simulink model "eclipse_target_lqri"  (Simulink 7.6)
settings: Solver=FixedStepDiscrete  StartTime=0.0  StopTime=inf  FixedStep=Ts  RelTol=1e-3
PreLoadFcn:
  | load_waypoints
values from neighbouring files (symbols this model uses):
  g = 9.8065    [kostas_malakies.mat]    (also in kostas_malakies2.mat; load_PMModel.m = 9.81; main.m; main_last.m)
  mass = 0.66    [kostas_malakies.mat]    (also in kostas_malakies2.mat; load_PMModel.m = 0.687; main_last.m)
  Ts = 0.02    [kostas_malakies.mat]    (also in kostas_malakies2.mat; main.m; main_last.m; matlab.mat = 0.08)
undefined symbols (not defined in the file or in its folder): DiscIntNeverNeededParam
libraries: Hquad_control_LIB_LQRI x13, Hqaud_model_LIB_SI x1, idelinklib_tgtpref x1, simulink x1
settings Model: Creator=janosch  LastModifiedBy=burrimi  SimulationMode=external
settings DataIOCC: SaveOutput=off  SaveTime=off
settings OptimizationCC: OptimizeModelRefInitCode=on  LifeSpan=1
settings DebuggingCC: ParameterPrecisionLossMsg=none
settings HardwareCC: ProdIntDivRoundTo=Zero  ProdEndianess=LittleEndian  ProdHWDeviceType=Intel Pentium
settings RTWCC: SystemTargetFile=idelink_ert.tlc  GenerateMakefile=off  TemplateMakefile=idelink_ert.tmf  Description=Embedded IDE Link ERT  ProcessScript=idelink_ert_make_rtw_hook
settings CodeAppCC: IgnoreCustomStorageClasses=off
settings ERTFactory: TargetFcnLib=ansi_tfl_table_tmw.mat  TargetFunctionLibrary=ANSI_C  UtilityFuncGeneration=Auto  ERTMultiwordTypeDef=System defined  ERTCodeCoverageTool=None  ERTMultiwordLength=256  MultiwordLength=2048  GenerateFullHeader=on  GenerateSampleERTMain=off  GenerateTestInterfaces=off  IsPILTarget=off  ModelReferenceCompliant=on  ParMdlRefBuildCompliant=off  CompOptLevelCompliant=off  IncludeMdlTerminateFcn=on  GeneratePreprocessorConditionals=Disable all  CombineOutputUpdateFcns=on  CombineSignalStateStructs=off  SuppressErrorStatus=off  ERTFirstTimeCompliant=off  IncludeFileDelimiter=Auto  ERTCustomFileBanners=on  SupportAbsoluteTime=on  LogVarNameModifier=rt_  MatFileLogging=off  MultiInstanceERTCode=off  SupportNonFinite=on  SupportComplex=on  PurelyIntegerCode=off  SupportContinuousTime=off  SupportNonInlinedSFcns=on  SupportVariableSizeSignals=off  EnableShiftOperators=on  ParenthesesLevel=Nominal  PortableWordSizes=off  ModelStepFunctionPrototypeControlCompliant=on  CPPClassGenCompliant=off  AutosarCompliant=off  GenerateErtSFunction=off  CreateSILPILBlock=None  GenerateASAP2=off  ExtMode=on  ExtModeTransport=0  ExtModeStaticAlloc=off  ExtModeStaticAllocSize=1000000  ExtModeTesting=off  ExtModeMexFile=ext_comm  ExtModeIntrfLevel=Level1  InlinedParameterPlacement=Hierarchical  TargetOS=BareBoardExample  MultiInstanceErrorCode=Error  RateGroupingCode=on  RootIOFormat=Individual arguments  RTWCAPISignals=off  RTWCAPIParams=off  RTWCAPIStates=off  ERTSrcFileBannerTemplate=ert_code_template.cgt  ERTHdrFileBannerTemplate=ert_code_template.cgt  ERTDataSrcFileTemplate=ert_code_template.cgt  ERTDataHdrFileTemplate=ert_code_template.cgt  ERTCustomFileTemplate=example_file_process.tlc  CoverageDialogOpen=off  ModuleNamingRule=Unspecified  SignalDisplayLevel=10  ParamTuneLevel=10  GlobalDataDefinition=Auto  DataDefinitionFile=global.c  GlobalDataReference=Auto  ERTFilePackagingFormat=Modular  DataReferenceFile=global.h  GRTInterface=off  PreserveExpressionOrder=off  PreserveIfCondition=off  ConvertIfToSwitch=off  PreserveExternInFcnDecls=on  EnableUserReplacementTypes=off  MemSecPackage=--- None ---  MemSecDataConstants=Default  MemSecDataIO=Default  MemSecDataInternal=Default  MemSecDataParameters=Default  MemSecFuncInitTerm=Default  MemSecFuncExecute=Default  AdaptorName=Eclipse  exportIDEObj=on  ideObjName=IDE_Obj  oldideObjName=IDE_Obj  ideObjTimeout=50  oldideObjTimeout=50  ideObjBuildTimeout=1000  oldideObjBuildTimeout=1000  ProfileGenCode=off  profileBy=Tasks  ProfileNumSamples=100  InlineDSPBlks=off  projectOptions=Custom  debugCompilerOptions="-g -D\"_DEBUG\""  releaseCompilerOptions=-O2  getCompilerOptions=off  resetCompilerOptions=off  debugLinkerOptions=-lm  releaseLinkerOptions=-lm  customLinkerOptions=-lm  linkerOptionsStr=-lm  getLinkerOptions=off  resetLinkerOptions=off  systemStackSize=512  systemHeapSize=512  buildFormat=Project  buildAction=Build  overrunNotificationMethod=None  overrunNotificationFcn=myfunction  oldoverrunNotificationFcn=myfunction  configurePIL=off  configPILBlockAction=Create_PIL_block_build_and_download  DiagnosticActions=warning

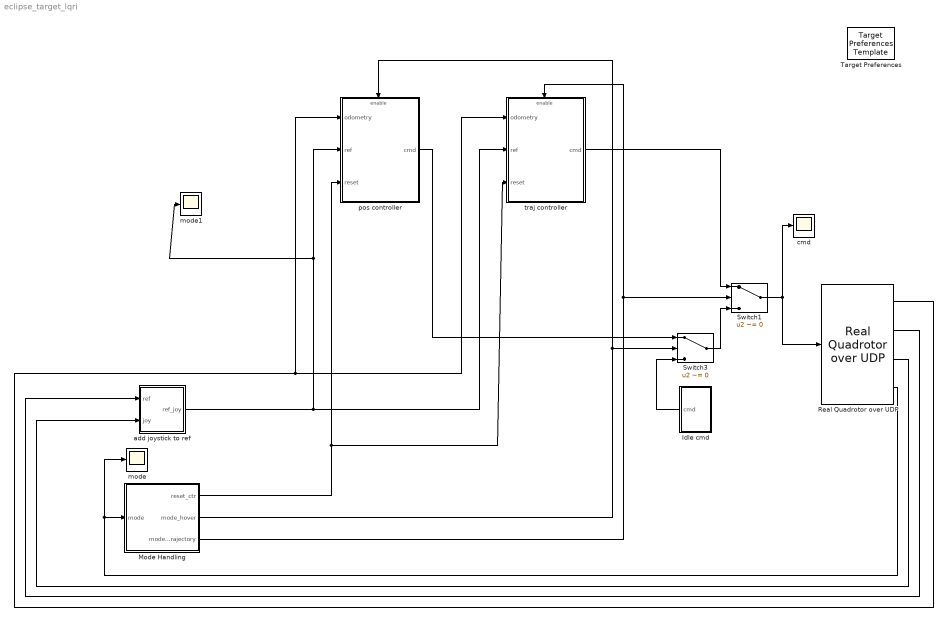
== system eclipse_target_lqri ==
  Idle cmd : Subsystem
  Mode Handling : Subsystem
  Real Quadrotor over UDP : Hqaud_model_LIB_SI/Real Quadrotor over UDP  SystemSampleTime=-1
  Switch1 : Switch  Criteria=u2 ~= 0
  Switch3 : Switch  Criteria=u2 ~= 0
  Target Preferences : idelinklib_tgtpref/Target Preferences Template  Tag=eclipseidetgtpref  SystemSampleTime=-1  library=off
  add joystick to ref : Subsystem
  cmd : Scope
      settings: YMin=-0.5  YMax=7  SaveName=ScopeData4
  mode : Scope
      settings: YMin=0  YMax=6  SaveName=ScopeData6
  mode1 : Scope
      settings: YMin=-2  YMax=2  SaveName=ScopeData7
  pos controller : Subsystem  AncestorBlock=Hquad_control_LIB_LQRI/pos controller
  traj controller : Subsystem  AncestorBlock=Hquad_control_LIB_LQRI/traj controller
  wires:
  Mode Handling/1(reset_ctr) -> pos controller/3(reset), traj controller/3(reset)
  Mode Handling/2(mode_hover) -> Switch3/2, pos controller/Enable
  Idle cmd/1(cmd) -> Switch3/3
  pos controller/1(cmd) -> Switch3/1
  Mode Handling/3(mode_trajectory) -> Switch1/2, traj controller/Enable
  Switch3/1 -> Switch1/3
  Switch1/1 -> cmd/1, Real Quadrotor over UDP/1
  traj controller/1(cmd) -> Switch1/1
  Real Quadrotor over UDP/3 -> add joystick to ref/2(joy)
  add joystick to ref/1(ref_joy) -> mode1/1, pos controller/2(ref), traj controller/2(ref)
  Real Quadrotor over UDP/2 -> add joystick to ref/1(ref)
  Real Quadrotor over UDP/1 -> pos controller/1(odometry), traj controller/1(odometry)
  Real Quadrotor over UDP/4 -> Mode Handling/1(mode), mode/1

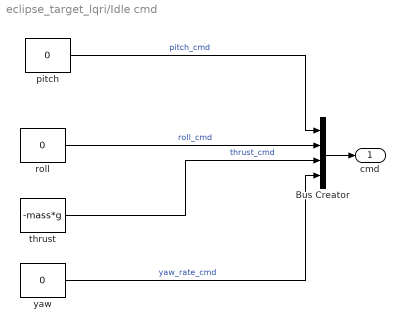
== system eclipse_target_lqri/Idle cmd ==
  Bus Creator : BusCreator
  pitch : Constant  Value=0
  roll : Constant  Value=0
  thrust : Constant  Value=-mass*g
  yaw : Constant  Value=0
  cmd : Outport
  wires:
  roll/1 -> Bus Creator/2  "roll_cmd"
  pitch/1 -> Bus Creator/1  "pitch_cmd"
  Bus Creator/1 -> cmd/1
  thrust/1 -> Bus Creator/3  "thrust_cmd"
  yaw/1 -> Bus Creator/4  "yaw_rate_cmd"

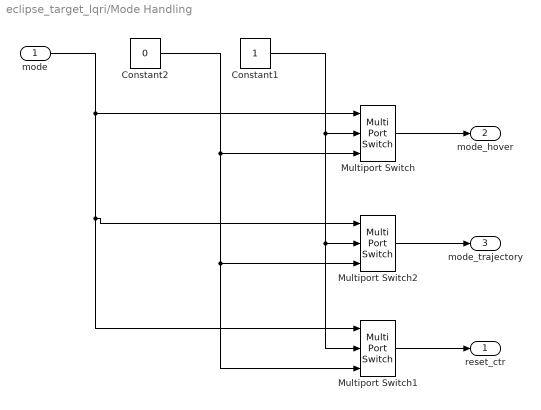
== system eclipse_target_lqri/Mode Handling ==
  mode : Inport
  Constant1 : Constant
  Constant2 : Constant  Value=0
  Multiport Switch : MultiPortSwitch  DataPortOrder=Specify indices  Inputs=2  DataPortIndices={[1,2,3],0}  zeroidx=off
  Multiport Switch1 : MultiPortSwitch  DataPortOrder=Specify indices  Inputs=2  DataPortIndices={[10],0}  zeroidx=off
  Multiport Switch2 : MultiPortSwitch  DataPortOrder=Specify indices  Inputs=2  DataPortIndices={[4],0}  zeroidx=off
  reset_ctr : Outport
  mode_hover : Outport  Port=2
  mode_trajectory : Outport  Port=3
  wires:
  Constant1/1 -> Multiport Switch/2, Multiport Switch1/2, Multiport Switch2/2
  Constant2/1 -> Multiport Switch/3, Multiport Switch1/3, Multiport Switch2/3
  Multiport Switch1/1 -> reset_ctr/1
  mode/1 -> Multiport Switch/1, Multiport Switch1/1, Multiport Switch2/1
  Multiport Switch/1 -> mode_hover/1
  Multiport Switch2/1 -> mode_trajectory/1

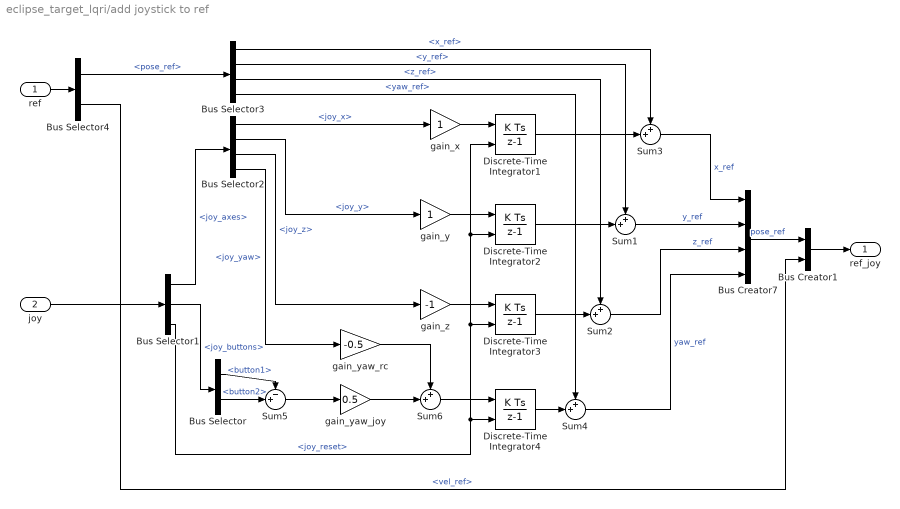
== system eclipse_target_lqri/add joystick to ref ==
  ref : Inport
  joy : Inport  Port=2
  Bus Creator1 : BusCreator  Inputs=2
  Bus Creator7 : BusCreator
  Bus Selector : BusSelector  OutputSignals=button1,button2
  Bus Selector1 : BusSelector  OutputSignals=joy_axes,joy_buttons,joy_reset
  Bus Selector2 : BusSelector  OutputSignals=joy_x,joy_y,joy_z,joy_yaw
  Bus Selector3 : BusSelector  OutputSignals=x_ref,y_ref,z_ref,yaw_ref
  Bus Selector4 : BusSelector  OutputSignals=pose_ref,vel_ref
  Discrete-Time Integrator{1..4} (4 alike) : DiscreteIntegrator  ExternalReset=rising  SampleTime=Ts  ICPrevOutput=DiscIntNeverNeededParam  ICPrevScaledInput=DiscIntNeverNeededParam
  Sum{1..4,6} (5 alike) : Sum  Inputs=++|
  Sum5 : Sum  Inputs=-+|
  gain_x : Gain
  gain_y : Gain
  gain_yaw_joy : Gain  Gain=0.5
  gain_yaw_rc : Gain  Gain=-0.5
  gain_z : Gain  Gain=-1
  ref_joy : Outport
  wires:
  Bus Selector2/1 -> gain_x/1  "<joy_x>"
  Bus Selector2/2 -> gain_y/1  "<joy_y>"
  Bus Selector2/3 -> gain_z/1  "<joy_z>"
  gain_x/1 -> Discrete-Time Integrator1/1
  gain_y/1 -> Discrete-Time Integrator2/1
  gain_z/1 -> Discrete-Time Integrator3/1
  Bus Selector3/1 -> Sum3/1  "<x_ref>"
  Bus Selector3/2 -> Sum1/1  "<y_ref>"
  Bus Selector3/3 -> Sum2/1  "<z_ref>"
  Discrete-Time Integrator1/1 -> Sum3/2
  Discrete-Time Integrator2/1 -> Sum1/2
  Discrete-Time Integrator3/1 -> Sum2/2
  Sum4/1 -> Bus Creator7/4  "yaw_ref"
  Sum2/1 -> Bus Creator7/3  "z_ref"
  Sum1/1 -> Bus Creator7/2  "y_ref"
  Sum3/1 -> Bus Creator7/1  "x_ref"
  Bus Selector1/2 -> Bus Selector/1  "<joy_buttons>"
  Bus Selector1/3 -> Discrete-Time Integrator3/2, Discrete-Time Integrator1/2, Discrete-Time Integrator2/2, Discrete-Time Integrator4/2  "<joy_reset>"
  Bus Selector/1 -> Sum5/1  "<button1>"
  Bus Selector/2 -> Sum5/2  "<button2>"
  Discrete-Time Integrator4/1 -> Sum4/2
  Bus Selector3/4 -> Sum4/1  "<yaw_ref>"
  joy/1 -> Bus Selector1/1
  Bus Selector1/1 -> Bus Selector2/1  "<joy_axes>"
  ref/1 -> Bus Selector4/1
  Bus Creator1/1 -> ref_joy/1
  Sum5/1 -> gain_yaw_joy/1
  Sum6/1 -> Discrete-Time Integrator4/1
  Bus Selector2/4 -> gain_yaw_rc/1  "<joy_yaw>"
  gain_yaw_rc/1 -> Sum6/1
  gain_yaw_joy/1 -> Sum6/2
  Bus Creator7/1 -> Bus Creator1/1  "pose_ref"
  Bus Selector4/1 -> Bus Selector3/1  "<pose_ref>"
  Bus Selector4/2 -> Bus Creator1/2  "<vel_ref>"

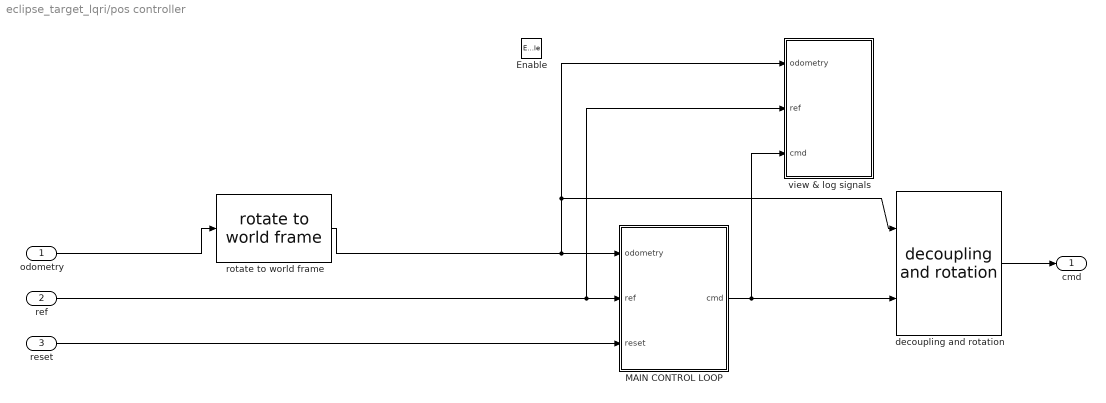
== system eclipse_target_lqri/pos controller ==
  odometry : Inport
  ref : Inport  Port=2
  reset : Inport  Port=3
  Enable : EnablePort  StatesWhenEnabling=reset
  MAIN CONTROL LOOP : Subsystem  AncestorBlock=Hquad_control_LIB_LQRI/MAIN CONTROL LOOP  TreatAsAtomicUnit=on
  decoupling and rotation : Hquad_control_LIB_LQRI/decoupling and rotation  Priority=3  SystemSampleTime=-1
  rotate to world frame : Hquad_control_LIB_LQRI/rotate to world frame  Priority=1  SystemSampleTime=-1
  view & log signals : Subsystem  AncestorBlock=Hquad_control_LIB_LQRI/view & log signals
  cmd : Outport
  wires:
  ref/1 -> MAIN CONTROL LOOP/2(ref), view & log signals/2(ref)
  reset/1 -> MAIN CONTROL LOOP/3(reset)
  odometry/1 -> rotate to world frame/1
  rotate to world frame/1 -> view & log signals/1(odometry), decoupling and rotation/1, MAIN CONTROL LOOP/1(odometry)
  MAIN CONTROL LOOP/1(cmd) -> view & log signals/3(cmd), decoupling and rotation/2
  decoupling and rotation/1 -> cmd/1

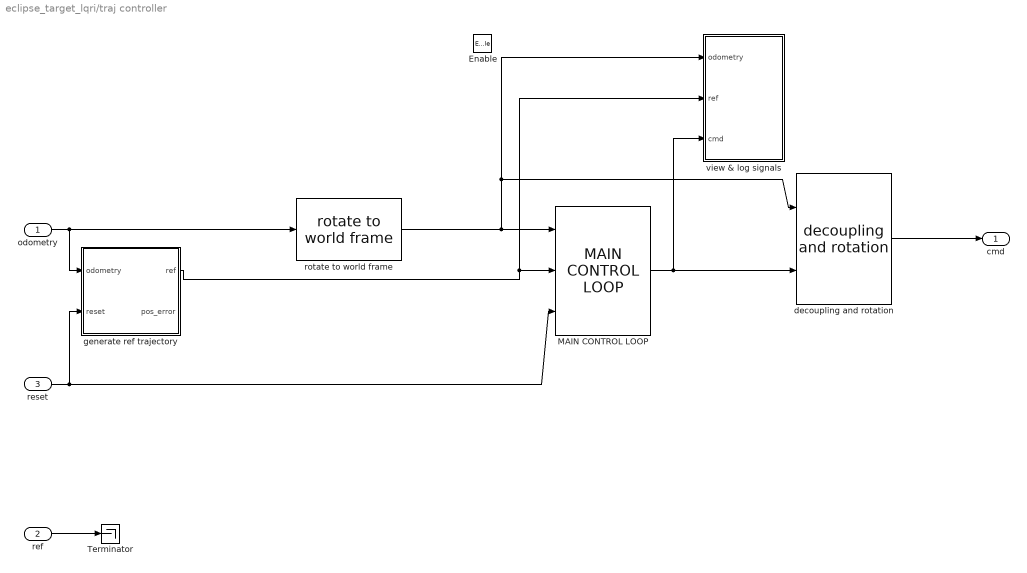
== system eclipse_target_lqri/traj controller ==
  odometry : Inport
  ref : Inport  Port=2
  reset : Inport  Port=3
  Enable : EnablePort  StatesWhenEnabling=reset
  MAIN CONTROL LOOP : Hquad_control_LIB_LQRI/MAIN CONTROL LOOP  SystemSampleTime=-1
  Terminator : Terminator
  decoupling and rotation : Hquad_control_LIB_LQRI/decoupling and rotation  Priority=3  SystemSampleTime=-1
  generate ref trajectory : Subsystem  AncestorBlock=Hquad_control_LIB_LQRI/generate ref trajectory
  rotate to world frame : Hquad_control_LIB_LQRI/rotate to world frame  Priority=1  SystemSampleTime=-1
  view & log signals : Subsystem  AncestorBlock=Hquad_control_LIB_LQRI/view & log signals
  cmd : Outport
  wires:
  generate ref trajectory/1(ref) -> MAIN CONTROL LOOP/2, view & log signals/2(ref)
  reset/1 -> MAIN CONTROL LOOP/3, generate ref trajectory/2(reset)
  ref/1 -> Terminator/1
  odometry/1 -> rotate to world frame/1, generate ref trajectory/1(odometry)
  rotate to world frame/1 -> view & log signals/1(odometry), decoupling and rotation/1, MAIN CONTROL LOOP/1
  MAIN CONTROL LOOP/1 -> view & log signals/3(cmd), decoupling and rotation/2
  decoupling and rotation/1 -> cmd/1

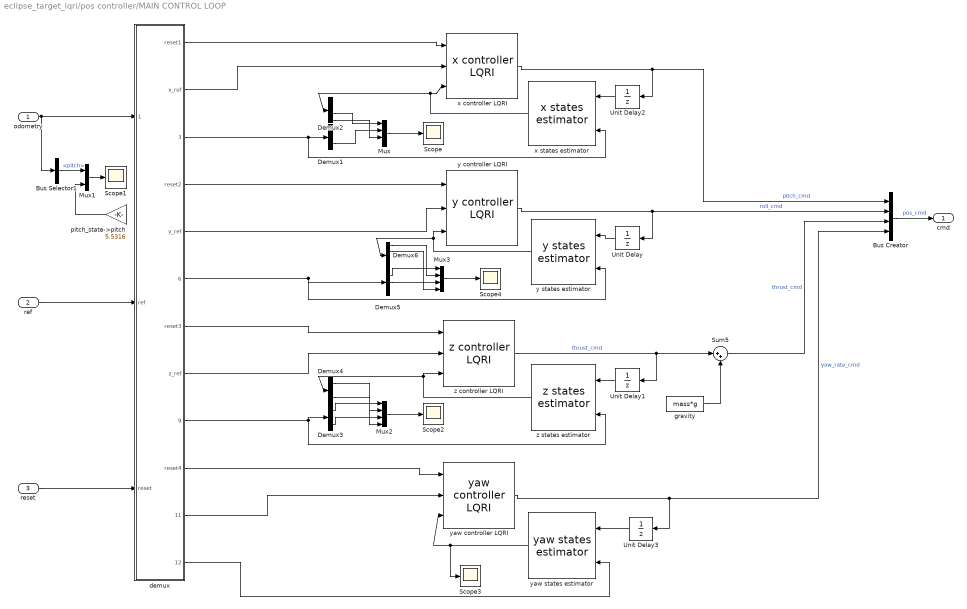
== system eclipse_target_lqri/pos controller/MAIN CONTROL LOOP ==
  odometry : Inport
  ref : Inport  Port=2
  reset : Inport  Port=3
  Bus Creator : BusCreator
  Bus Selector1 : BusSelector  OutputSignals=rpy.pitch
  Demux1 : Demux  Outputs=3
  Demux2 : Demux
  Demux3 : Demux  Outputs=2
  Demux4 : Demux  Outputs=2
  Demux5 : Demux  Outputs=3
  Demux6 : Demux
  Mux : Mux
  Mux1 : Mux  Inputs=2
  Mux2 : Mux
  Mux3 : Mux
  Scope{,1..4} (5 alike) : Scope
      Scope settings: TimeRange=8.564360869565219  YMin=-50  YMax=2.5  SaveName=ScopeData13
      Scope1 settings: YMin=-0.4  YMax=1.4  SaveName=ScopeData14
      Scope2 settings: YMin=-1.5  YMax=0.4  SaveName=ScopeData15
      Scope3 settings: YMin=-0.03  YMax=0.09  SaveName=ScopeData16
      Scope4 settings: TimeRange=8.564360869565219  YMin=-0.2  YMax=2  SaveName=ScopeData4
  Sum5 : Sum  Inputs=|++
  Unit Delay{,1..3} (4 alike) : UnitDelay  SampleTime=Ts
  demux : Subsystem
  gravity : Constant  Value=mass*g
  pitch_state->pitch : Gain  Gain=5.5316
  "x controller LQRI  " : Hquad_control_LIB_LQRI/x controller LQRI    SystemSampleTime=-1
  x states estimator : Hquad_control_LIB_LQRI/x states estimator  SystemSampleTime=-1
  y controller LQRI : Hquad_control_LIB_LQRI/y controller LQRI  SystemSampleTime=-1
  y states estimator : Hquad_control_LIB_LQRI/y states estimator  SystemSampleTime=-1
  yaw controller LQRI : Hquad_control_LIB_LQRI/yaw controller LQRI  SystemSampleTime=-1
  yaw states estimator : Hquad_control_LIB_LQRI/yaw states estimator  SystemSampleTime=-1
  z controller LQRI : Hquad_control_LIB_LQRI/z controller LQRI  SystemSampleTime=-1
  z states estimator : Hquad_control_LIB_LQRI/z states estimator  SystemSampleTime=-1
  cmd : Outport
  wires:
  Unit Delay3/1 -> yaw states estimator/1
  Sum5/1 -> Bus Creator/3  "thrust_cmd"
  demux/11(yaw_ref) -> yaw controller LQRI/2
  demux/9(z_states_meas) -> z states estimator/2, Demux3/1
  demux/6(y_states_meas) -> y states estimator/2, Demux5/1
  demux/3(x_states_meas) -> x states estimator/2, Demux1/1
  Bus Creator/1 -> cmd/1  "pos_cmd"
  demux/10(reset4) -> yaw controller LQRI/1
  demux/1(reset1) -> "x controller LQRI  "/1
  reset/1 -> demux/3(reset)
  ref/1 -> demux/2(ref)
  odometry/1 -> demux/1(odometry), Bus Selector1/1
  yaw controller LQRI/1 -> Unit Delay3/1, Bus Creator/4  "yaw_rate_cmd"
  demux/12(yaw_states_meas) -> yaw states estimator/2
  Unit Delay2/1 -> x states estimator/1
  Unit Delay1/1 -> z states estimator/1
  Unit Delay/1 -> y states estimator/1
  demux/2(x_ref) -> "x controller LQRI  "/2
  x states estimator/1 -> "x controller LQRI  "/3, Demux2/1
  y states estimator/1 -> y controller LQRI/3, Demux6/1
  "x controller LQRI  "/1 -> Unit Delay2/1, Bus Creator/1  "pitch_cmd"
  y controller LQRI/1 -> Unit Delay/1, Bus Creator/2  "roll_cmd"
  z states estimator/1 -> z controller LQRI/3, Demux4/1
  Mux/1 -> Scope/1
  Mux1/1 -> Scope1/1
  Bus Selector1/1 -> Mux1/1  "<pitch>"
  pitch_state->pitch/1 -> Mux1/2
  Mux2/1 -> Scope2/1
  Demux3/1 -> Mux2/1
  Demux4/1 -> Mux2/2
  Demux3/2 -> Mux2/3
  z controller LQRI/1 -> Unit Delay1/1, Sum5/1  "thrust_cmd"
  yaw states estimator/1 -> yaw controller LQRI/3, Scope3/1
  gravity/1 -> Sum5/2
  demux/5(y_ref) -> y controller LQRI/2
  demux/4(reset2) -> y controller LQRI/1
  Mux3/1 -> Scope4/1
  Demux5/1 -> Mux3/1
  Demux6/1 -> Mux3/2
  Demux5/2 -> Mux3/3
  Demux6/2 -> Mux3/4
  Demux4/2 -> Mux2/4
  demux/8(z_ref) -> z controller LQRI/2
  demux/7(reset3) -> z controller LQRI/1
  Demux2/3 -> Mux/1
  Demux1/3 -> Mux/2
  Demux2/4 -> Mux/3

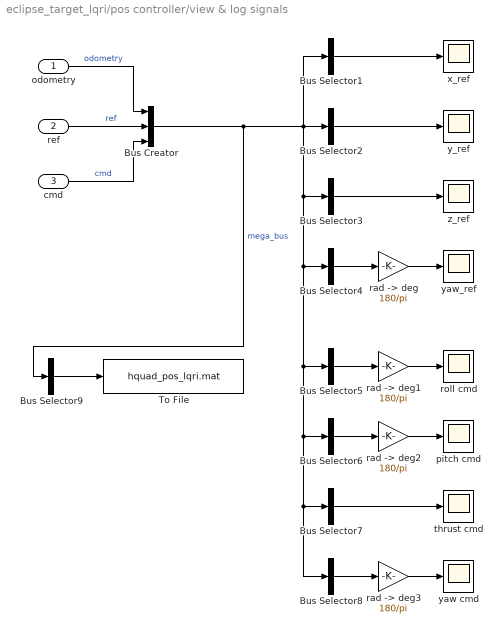
== system eclipse_target_lqri/pos controller/view & log signals ==
  odometry : Inport
  ref : Inport  Port=2
  cmd : Inport  Port=3
  Bus Creator : BusCreator  Inputs=3
  Bus Selector1 : BusSelector  OutputSignals=odometry.pos.x,odometry.vel.x_dot,ref.pose_ref.x_ref,ref.vel_ref.x_dot_ref  OutputAsBus=on
  Bus Selector2 : BusSelector  OutputSignals=odometry.pos.y,odometry.vel.y_dot,ref.pose_ref.y_ref,ref.vel_ref.y_dot_ref  OutputAsBus=on
  Bus Selector3 : BusSelector  OutputSignals=odometry.pos.z,odometry.vel.z_dot,ref.pose_ref.z_ref,ref.vel_ref.z_dot_ref  OutputAsBus=on
  Bus Selector4 : BusSelector  OutputSignals=odometry.rpy.yaw,odometry.ang_vel.ang_vel_z,ref.pose_ref.yaw_ref,ref.vel_ref.yaw_dot_ref  OutputAsBus=on
  Bus Selector5 : BusSelector  OutputSignals=odometry.rpy.roll,odometry.ang_vel.ang_vel_x,cmd.roll_cmd  OutputAsBus=on
  Bus Selector6 : BusSelector  OutputSignals=odometry.rpy.pitch,odometry.ang_vel.ang_vel_y,cmd.pitch_cmd  OutputAsBus=on
  Bus Selector7 : BusSelector  OutputSignals=odometry.pos.z,ref.pose_ref.z_ref,cmd.thrust_cmd  OutputAsBus=on
  Bus Selector8 : BusSelector  OutputSignals=odometry.rpy.yaw,odometry.ang_vel.ang_vel_z,cmd.yaw_rate_cmd  OutputAsBus=on
  Bus Selector9 : BusSelector  OutputSignals=odometry.pos.x,odometry.vel.x_dot,odometry.rpy.pitch,ref.pose_ref.x_ref,cmd.pitch_cmd,odometry.pos.y,odometry.vel.y_dot,odometry.rpy.roll,ref.pose_ref.y_ref,cmd.roll_cmd,odometry.pos.z,odometry.vel.z_dot,ref.pose_ref.z_ref,cmd.thrust_cmd,odometry.rpy.yaw,odometry.ang_vel.ang_vel_z,ref.pose_ref.yaw_ref,cmd.yaw_rate_cmd  OutputAsBus=on
  To File : ToFile  Filename=hquad_pos_lqri.mat  MatrixName=hquad_pos_lqri
  pitch cmd : Scope
      settings: YMin=-15  YMax=15  SaveName=ScopeData2
  rad -> deg{,1..3} (4 alike) : Gain  Gain=180/pi
  roll cmd : Scope
      settings: YMin=-100  YMax=100
  thrust cmd : Scope
      settings: YMin=-3  YMax=3  SaveName=ScopeData11
  x_ref : Scope
      settings: TimeRange=40  YMin=-0.8  YMax=0.9  SaveName=ScopeData3
  y_ref : Scope
      settings: TimeRange=40  YMin=-0.2  YMax=2.1
  yaw cmd : Scope
      settings: YMin=-60  YMax=-0  SaveName=ScopeData10
  yaw_ref : Scope
      settings: TimeRange=39.996  YMin=0  YMax=3250  SaveName=ScopeData8
  z_ref : Scope
      settings: YMin=-1.2  YMax=0.1  SaveName=ScopeData5
  wires:
  Bus Selector9/1 -> To File/1
  "rad -> deg"/1 -> yaw_ref/1
  "rad -> deg1"/1 -> roll cmd/1
  "rad -> deg2"/1 -> pitch cmd/1
  "rad -> deg3"/1 -> yaw cmd/1
  odometry/1 -> Bus Creator/1  "odometry"
  ref/1 -> Bus Creator/2  "ref"
  cmd/1 -> Bus Creator/3  "cmd"
  Bus Creator/1 -> Bus Selector9/1, Bus Selector1/1, Bus Selector2/1, Bus Selector3/1, Bus Selector4/1, Bus Selector5/1, Bus Selector6/1, Bus Selector7/1, Bus Selector8/1  "mega_bus"
  Bus Selector1/1 -> x_ref/1
  Bus Selector2/1 -> y_ref/1
  Bus Selector3/1 -> z_ref/1
  Bus Selector4/1 -> "rad -> deg"/1
  Bus Selector7/1 -> thrust cmd/1
  Bus Selector5/1 -> "rad -> deg1"/1
  Bus Selector6/1 -> "rad -> deg2"/1
  Bus Selector8/1 -> "rad -> deg3"/1

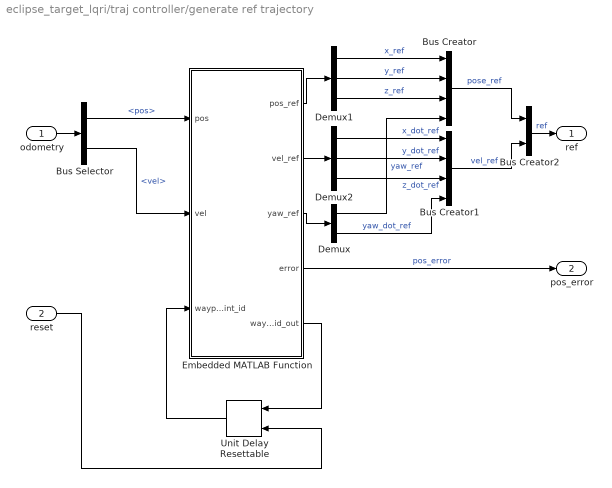
== system eclipse_target_lqri/traj controller/generate ref trajectory ==
  odometry : Inport
  reset : Inport  Port=2
  Bus Creator : BusCreator
  Bus Creator1 : BusCreator
  Bus Creator2 : BusCreator  Inputs=2
  Bus Selector : BusSelector  OutputSignals=pos,vel
  Demux : Demux  Outputs=2
  Demux1 : Demux  Outputs=3
  Demux2 : Demux  Outputs=3
  Embedded MATLAB Function : Stateflow chart  TreatAsAtomicUnit=on
  Unit Delay Resettable : simulink/Additional Math & Discrete/Additional Discrete/Unit Delay Resettable  SystemSampleTime=-1  vinit=0.0  tsamp=-1
  ref : Outport
  pos_error : Outport  Port=2
  wires:
  Bus Selector/2 -> Embedded MATLAB Function/2(vel)  "<vel>"
  Bus Selector/1 -> Embedded MATLAB Function/1(pos)  "<pos>"
  odometry/1 -> Bus Selector/1
  Unit Delay Resettable/1 -> Embedded MATLAB Function/3(waypoint_id)
  Embedded MATLAB Function/5(waypoint_id_out) -> Unit Delay Resettable/1
  Embedded MATLAB Function/3(yaw_ref) -> Demux/1
  Embedded MATLAB Function/4(error) -> pos_error/1  "pos_error"
  Embedded MATLAB Function/1(pos_ref) -> Demux1/1
  Embedded MATLAB Function/2(vel_ref) -> Demux2/1
  Demux1/1 -> Bus Creator/1  "x_ref"
  Demux1/2 -> Bus Creator/2  "y_ref"
  Demux1/3 -> Bus Creator/3  "z_ref"
  Demux/1 -> Bus Creator/4  "yaw_ref"
  Demux2/1 -> Bus Creator1/1  "x_dot_ref"
  Demux2/2 -> Bus Creator1/2  "y_dot_ref"
  Demux2/3 -> Bus Creator1/3  "z_dot_ref"
  Demux/2 -> Bus Creator1/4  "yaw_dot_ref"
  Bus Creator/1 -> Bus Creator2/1  "pose_ref"
  Bus Creator1/1 -> Bus Creator2/2  "vel_ref"
  reset/1 -> Unit Delay Resettable/2
  Bus Creator2/1 -> ref/1  "ref"

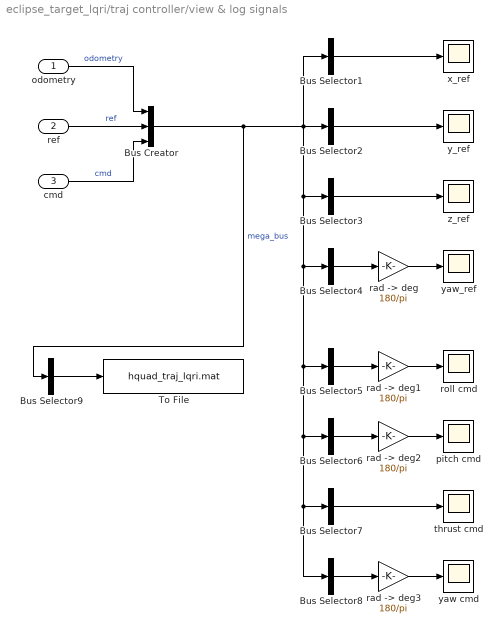
== system eclipse_target_lqri/traj controller/view & log signals ==
  odometry : Inport
  ref : Inport  Port=2
  cmd : Inport  Port=3
  Bus Creator : BusCreator  Inputs=3
  Bus Selector1 : BusSelector  OutputSignals=odometry.pos.x,odometry.vel.x_dot,ref.pose_ref.x_ref,ref.vel_ref.x_dot_ref  OutputAsBus=on
  Bus Selector2 : BusSelector  OutputSignals=odometry.pos.y,odometry.vel.y_dot,ref.pose_ref.y_ref,ref.vel_ref.y_dot_ref  OutputAsBus=on
  Bus Selector3 : BusSelector  OutputSignals=odometry.pos.z,odometry.vel.z_dot,ref.pose_ref.z_ref,ref.vel_ref.z_dot_ref  OutputAsBus=on
  Bus Selector4 : BusSelector  OutputSignals=odometry.rpy.yaw,odometry.ang_vel.ang_vel_z,ref.pose_ref.yaw_ref,ref.vel_ref.yaw_dot_ref  OutputAsBus=on
  Bus Selector5 : BusSelector  OutputSignals=odometry.rpy.roll,odometry.ang_vel.ang_vel_x,cmd.roll_cmd  OutputAsBus=on
  Bus Selector6 : BusSelector  OutputSignals=odometry.rpy.pitch,odometry.ang_vel.ang_vel_y,cmd.pitch_cmd  OutputAsBus=on
  Bus Selector7 : BusSelector  OutputSignals=odometry.pos.z,ref.pose_ref.z_ref,cmd.thrust_cmd  OutputAsBus=on
  Bus Selector8 : BusSelector  OutputSignals=odometry.rpy.yaw,odometry.ang_vel.ang_vel_z,cmd.yaw_rate_cmd  OutputAsBus=on
  Bus Selector9 : BusSelector  OutputSignals=odometry.pos.x,odometry.vel.x_dot,odometry.rpy.pitch,ref.pose_ref.x_ref,cmd.pitch_cmd,odometry.pos.y,odometry.vel.y_dot,odometry.rpy.roll,ref.pose_ref.y_ref,cmd.roll_cmd,odometry.pos.z,odometry.vel.z_dot,ref.pose_ref.z_ref,cmd.thrust_cmd,odometry.rpy.yaw,odometry.ang_vel.ang_vel_z,ref.pose_ref.yaw_ref,cmd.yaw_rate_cmd  OutputAsBus=on
  To File : ToFile  Filename=hquad_traj_lqri.mat  MatrixName=hquad_traj_lqri
  pitch cmd : Scope
      settings: YMin=-15  YMax=15  SaveName=ScopeData2
  rad -> deg{,1..3} (4 alike) : Gain  Gain=180/pi
  roll cmd : Scope
      settings: YMin=-100  YMax=100
  thrust cmd : Scope
      settings: YMin=-3  YMax=3  SaveName=ScopeData11
  x_ref : Scope
      settings: TimeRange=40  YMin=-1.5  YMax=1.5  SaveName=ScopeData3
  y_ref : Scope
      settings: TimeRange=40  YMin=-1.5  YMax=1.5
  yaw cmd : Scope
      settings: YMin=-60  YMax=-0  SaveName=ScopeData10
  yaw_ref : Scope
      settings: TimeRange=39.996  YMin=0  YMax=3250  SaveName=ScopeData8
  z_ref : Scope
      settings: YMin=-0.05  YMax=1.05  SaveName=ScopeData5
  wires:
  Bus Selector9/1 -> To File/1
  "rad -> deg"/1 -> yaw_ref/1
  "rad -> deg1"/1 -> roll cmd/1
  "rad -> deg2"/1 -> pitch cmd/1
  "rad -> deg3"/1 -> yaw cmd/1
  odometry/1 -> Bus Creator/1  "odometry"
  ref/1 -> Bus Creator/2  "ref"
  cmd/1 -> Bus Creator/3  "cmd"
  Bus Creator/1 -> Bus Selector9/1, Bus Selector1/1, Bus Selector2/1, Bus Selector3/1, Bus Selector4/1, Bus Selector5/1, Bus Selector6/1, Bus Selector7/1, Bus Selector8/1  "mega_bus"
  Bus Selector1/1 -> x_ref/1
  Bus Selector2/1 -> y_ref/1
  Bus Selector3/1 -> z_ref/1
  Bus Selector4/1 -> "rad -> deg"/1
  Bus Selector7/1 -> thrust cmd/1
  Bus Selector5/1 -> "rad -> deg1"/1
  Bus Selector6/1 -> "rad -> deg2"/1
  Bus Selector8/1 -> "rad -> deg3"/1

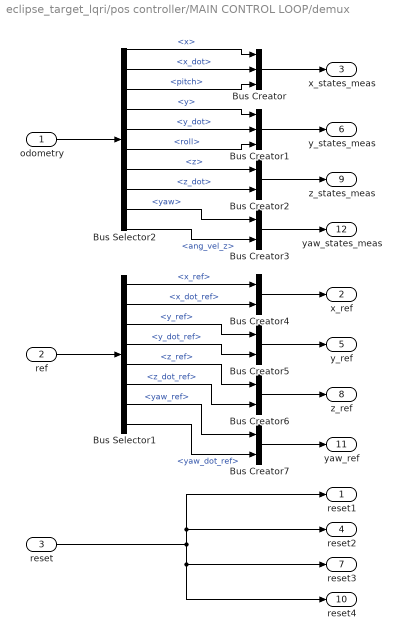
== system eclipse_target_lqri/pos controller/MAIN CONTROL LOOP/demux ==
  odometry : Inport
  ref : Inport  Port=2
  reset : Inport  Port=3
  Bus Creator : BusCreator  Inputs=3
  Bus Creator1 : BusCreator  Inputs=3
  Bus Creator{2..7} (6 alike) : BusCreator  Inputs=2
  Bus Selector1 : BusSelector  OutputSignals=pose_ref.x_ref,vel_ref.x_dot_ref,pose_ref.y_ref,vel_ref.y_dot_ref,pose_ref.z_ref,vel_ref.z_dot_ref,pose_ref.yaw_ref,vel_ref.yaw_dot_ref
  Bus Selector2 : BusSelector  OutputSignals=pos.x,vel.x_dot,rpy.pitch,pos.y,vel.y_dot,rpy.roll,pos.z,vel.z_dot,rpy.yaw,ang_vel.ang_vel_z
  reset1 : Outport
  x_ref : Outport  Port=2  PortDimensions=2
  x_states_meas : Outport  Port=3  PortDimensions=3
  reset2 : Outport  Port=4
  y_ref : Outport  Port=5  PortDimensions=2
  y_states_meas : Outport  Port=6  PortDimensions=3
  reset3 : Outport  Port=7
  z_ref : Outport  Port=8  PortDimensions=2
  z_states_meas : Outport  Port=9  PortDimensions=2
  reset4 : Outport  Port=10
  yaw_ref : Outport  Port=11  PortDimensions=2
  yaw_states_meas : Outport  Port=12  PortDimensions=2
  wires:
  reset/1 -> reset1/1, reset2/1, reset4/1, reset3/1
  Bus Selector1/8 -> Bus Creator7/2  "<yaw_dot_ref>"
  Bus Selector1/7 -> Bus Creator7/1  "<yaw_ref>"
  Bus Selector1/6 -> Bus Creator6/2  "<z_dot_ref>"
  Bus Selector1/5 -> Bus Creator6/1  "<z_ref>"
  Bus Selector1/4 -> Bus Creator5/2  "<y_dot_ref>"
  Bus Selector1/3 -> Bus Creator5/1  "<y_ref>"
  Bus Selector1/2 -> Bus Creator4/2  "<x_dot_ref>"
  Bus Creator4/1 -> x_ref/1
  Bus Creator5/1 -> y_ref/1
  Bus Creator6/1 -> z_ref/1
  Bus Creator7/1 -> yaw_ref/1
  Bus Selector1/1 -> Bus Creator4/1  "<x_ref>"
  ref/1 -> Bus Selector1/1
  Bus Creator3/1 -> yaw_states_meas/1
  Bus Creator2/1 -> z_states_meas/1
  Bus Selector2/10 -> Bus Creator3/2  "<ang_vel_z>"
  Bus Selector2/9 -> Bus Creator3/1  "<yaw>"
  Bus Selector2/8 -> Bus Creator2/2  "<z_dot>"
  Bus Selector2/7 -> Bus Creator2/1  "<z>"
  Bus Creator1/1 -> y_states_meas/1
  Bus Selector2/5 -> Bus Creator1/2  "<y_dot>"
  Bus Selector2/4 -> Bus Creator1/1  "<y>"
  Bus Selector2/2 -> Bus Creator/2  "<x_dot>"
  Bus Selector2/1 -> Bus Creator/1  "<x>"
  Bus Creator/1 -> x_states_meas/1
  odometry/1 -> Bus Selector2/1
  Bus Selector2/3 -> Bus Creator/3  "<pitch>"
  Bus Selector2/6 -> Bus Creator1/3  "<roll>"

== matlab function traj controller/generate ref trajectory/Embedded MATLAB Function ==
  data: pos input double; pos_ref output double; vel input double; vel_ref output double; yaw_ref output double; error output double; waypoint_id input double; waypoint_id_out output double
function [pos_ref,vel_ref,yaw_ref,error,waypoint_id_out] = fcn(pos,vel,waypoint_id)
%#eml

% speed=1;
% yaw=0;

% set how fast the quadrokopter flies to first waypoint
speed_init=0.5;

% waypoints=[0,0,-1;
%         -0.5,-1,-1;
%         0.5,-0.5,-1;
%         -0.5,-0.5,-1;
%         0.5,-1,-1;
%         0,0,-1];

% waypoints = [0, 0, -1, yaw, speed;
%     0, -1, -1, yaw, speed;
%     1, -1, -1, yaw, speed;
%     1, 0, -1, yaw, speed;
%     0, 0, -1, yaw, speed;
%     0, -1, -1, yaw, speed;
%     1, -1, -1, yaw, speed;
%     1, 0, -1, yaw, speed;
%     0, 0, -1, yaw, speed;
%     ];

speed=0.5;
yaw=-2.35619449;


waypoints = [2, -0.4, -1, yaw, speed;
    2, -1.4, -1, yaw, speed;
    1, -1.4, -1, yaw, speed;
    1, -0.4, -1, yaw, speed;
    2, -0.4, -1, yaw, speed;
    2, -1.4, -1, yaw, speed;
    1, -1.4, -1, yaw, speed;
    1, -0.4, -1, yaw, speed;
    2, -0.4, -1, yaw, speed;
    ];



num_waypoints=size(waypoints,1);
    


%i=dsearchn(waypoints,Pos);
% d=(waypoints(:,1)-Pos(1)).^2+(waypoints(:,2)-Pos(2)).^2+(waypoints(:,3)-Pos(3)).^2
% [V,i]=min(d);
% 
% if waypoint_id~=num_waypoints && waypoint_id~=1
%     if norm(waypoints(waypoint_id-1,:)-Pos)>norm(waypoints(waypoint_id+1,:)-Pos)
%         waypoint_id=waypoint_id+1;
%     end
% end


if waypoint_id~=num_waypoints
    if waypoint_id~=0
        P1=waypoints(waypoint_id,1:3)';
        yaw1=waypoints(waypoint_id,4);
        speed=waypoints(waypoint_id,5);
    else
        P1=pos;
        % set yaw ref to ref of first waypoint
        yaw1=waypoints(1,4);
        speed=speed_init;
    end
%     P1=waypoints(waypoint_id,:)';
    P2=waypoints(waypoint_id+1,1:3)';
    yaw2=waypoints(waypoint_id+1,4);
    
    %derive vector between two waypoints
    v=(P2-P1);
    if norm(v)==0   %if 2 waypoint are equal just skip to next waypoint
        waypoint_id=waypoint_id+1;
        pos_ref=pos;
        yaw_ref=[yaw1;0];
        vel_ref=[0,0,0]';
    else
        t=(pos-P1)'*v/(v'*v);
        pos_ref=P1+t*v;
        yaw_ref=[yaw1+t*(yaw2-yaw1);0];
        % set reference velocity
        vel_ref=v/norm(v)*speed;

        % fly slower depending on the distance error from the reference
        dist_error=norm(pos_ref-pos);
        vel_ref=vel_ref*(1-dist_error*1/0.3);
        
        % set next waypoint if close enough
        if norm(pos_ref-P2)<0.05 || t>1
            waypoint_id=waypoint_id+1;
        end
    end
else %stay at the last waypoint
    pos_ref=waypoints(waypoint_id,1:3)';
    yaw_ref=[waypoints(waypoint_id,4); 0];
    vel_ref=[0,0,0]';
end

error=[norm(pos_ref-pos);norm(vel_ref-vel)];


waypoint_id_out=waypoint_id;
